simulink model "RBD_Adjoint"  (R2022a)
settings: Solver=ode4  StartTime=0.0  StopTime=10  FixedStep=0.001  MaxStep=0.01  RelTol=1e-3
model workspace (MAT data in the model file):
  D = 2
  K = 2
  X_d = [5; 5; 5]
values from neighbouring files (symbols this model uses):
  Ic = 2.0 0.0 0.0 0.0 5.0 0.0 0.0 0.0 8.0    [dictionary.sldd]
  m = 2.0    [dictionary.sldd]
  v_0 = 2.0 0.0 0.0    [dictionary.sldd]
  w_0 = 0.0 0.0 0.0    [dictionary.sldd]
settings Model: DataDictionary=dictionary.sldd  Creator=Tommaso  LastModifiedBy=Tommaso
settings OptimizationCC: DefaultParameterBehavior=Inlined  UseDivisionForNetSlopeComputation=on  GainParamInheritBuiltInType=on  UseFloatMulNetSlope=on  InlineInvariantSignals=on  PassReuseOutputArgsThreshold=0  ZeroExternalMemoryAtStartup=off  ZeroInternalMemoryAtStartup=off  EfficientFloat2IntCast=on  OptimizeBlockOrder=speed  DifferentSizesBufferReuse=on
settings DebuggingCC: ParameterTunabilityLossMsg=error  BusObjectLabelMismatch=error
settings SFSimCC: MATLABDynamicMemAlloc=off
settings RTWCC: Description=Generic Real-Time Target  GenerateReport=on  LaunchReport=on  TargetLang=C++
settings CodeAppCC: ForceParamTrailComments=on  OperatorAnnotations=on
settings GRTTargetCC: TargetLangStandard=C++11 (ISO)  CodeInterfacePackaging=C++ class  MultiInstanceErrorCode=Warning

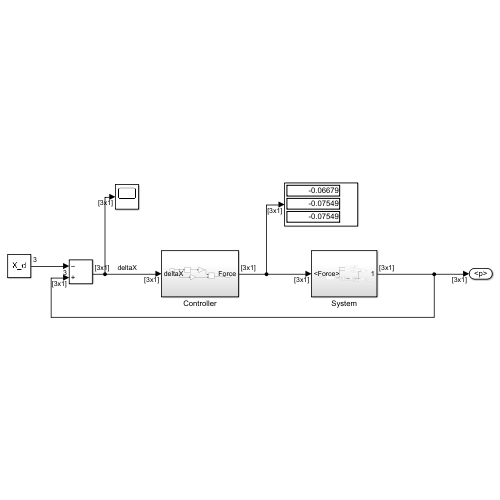
[thumbnail: Simulink's stored preview of the top-level diagram]
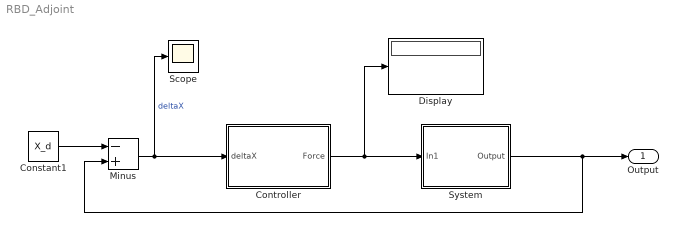
== system RBD_Adjoint ==
  Constant1 : Constant  Value=X_d
  Controller : Subsystem
  Display : Display
  Minus : Sum  Inputs=-+
  Scope : Scope
  System : Subsystem
  Output : Outport
  wires:
  System/1(Output) -> Output/1, Minus/2
  Constant1/1 -> Minus/1
  Minus/1 -> Controller/1(deltaX), Scope/1  "deltaX"
  Controller/1(Force) -> System/1(In1), Display/1

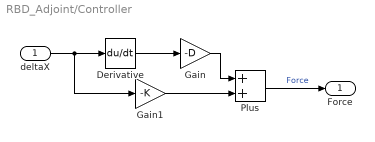
== system RBD_Adjoint/Controller ==
  deltaX : Inport
  Derivative : Derivative
  Gain : Gain  Gain=-D
  Gain1 : Gain  Gain=-K
  Plus : Sum
  Force : Outport
  wires:
  Derivative/1 -> Gain/1
  Gain1/1 -> Plus/2
  Gain/1 -> Plus/1
  Plus/1 -> Force/1  "Force"
  deltaX/1 -> Gain1/1, Derivative/1

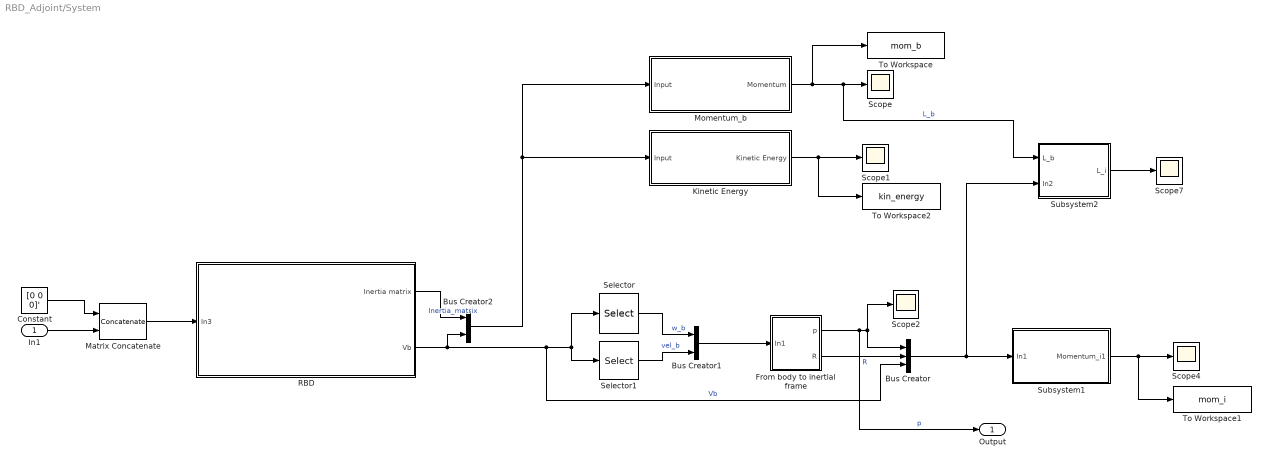
== system RBD_Adjoint/System ==
  In1 : Inport
  Bus Creator : BusCreator  Inputs=3  OutDataTypeStr=Bus: R_p_Vb
  Bus Creator1 : BusCreator  Inputs=2  OutDataTypeStr=Bus: Vb_bus  NonVirtualBus=on
  Bus Creator2 : BusCreator  Inputs=2  OutDataTypeStr=Bus: Inertia_Vb
  Constant : Constant  Value=[0 0 0]'
  From body to inertial frame : Subsystem  TreatAsAtomicUnit=on
  Kinetic Energy : Subsystem  TreatAsAtomicUnit=on
  Matrix Concatenate : Concatenate  Mode=Multidimensional array
  Momentum_b : Subsystem  TreatAsAtomicUnit=on
  RBD : Subsystem  TreatAsAtomicUnit=on
  Scope{,1..2,4,7} (5 alike) : Scope
  Selector : Selector  InputPortWidth=6  IndexOptions=Index vector (dialog)  Indices=[1,2,3]  OutputSizes=1
  Selector1 : Selector  InputPortWidth=6  IndexOptions=Index vector (dialog)  Indices=[4:6]  OutputSizes=1
  Subsystem1 : Subsystem  TreatAsAtomicUnit=on
  Subsystem2 : Subsystem  TreatAsAtomicUnit=on
  To Workspace : ToWorkspace  VariableName=mom_b  SampleTime=-1
  To Workspace1 : ToWorkspace  VariableName=mom_i  SampleTime=-1
  To Workspace2 : ToWorkspace  VariableName=kin_energy  SampleTime=-1
  Output : Outport
  wires:
  Subsystem1/1(Momentum_i1) -> To Workspace1/1, Scope4/1
  Bus Creator/1 -> Subsystem1/1(In1), Subsystem2/2(In2)
  Momentum_b/1(Momentum) -> To Workspace/1, Subsystem2/1(L_b), Scope/1  "L_b"
  Selector/1 -> Bus Creator1/1  "w_b"
  Kinetic Energy/1(Kinetic Energy) -> To Workspace2/1, Scope1/1
  RBD/1(Inertia matrix) -> Bus Creator2/1  "Inertia_matrix"
  Bus Creator2/1 -> Momentum_b/1(Input), Kinetic Energy/1(Input)
  Selector1/1 -> Bus Creator1/2  "vel_b"
  RBD/2(Vb) -> Bus Creator2/2, Bus Creator/3, Selector/1, Selector1/1  "Vb"
  Bus Creator1/1 -> From body to inertial frame/1(In1)
  From body to inertial frame/1(p) -> Output/1, Bus Creator/1, Scope2/1  "p"
  From body to inertial frame/2(R) -> Bus Creator/2  "R"
  Subsystem2/1(L_i) -> Scope7/1
  In1/1 -> Matrix Concatenate/2
  Matrix Concatenate/1 -> RBD/1(In3)
  Constant/1 -> Matrix Concatenate/1

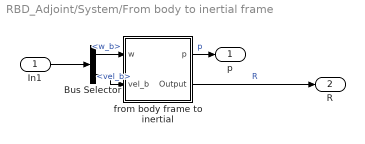
== system RBD_Adjoint/System/From body to inertial frame ==
  In1 : Inport
  Bus Selector : BusSelector  OutputSignals=w_b,vel_b
  from body frame to inertial : Subsystem
  p : Outport
  R : Outport  Port=2
  wires:
  Bus Selector/1 -> from body frame to inertial/1(w)  "<w_b>"
  from body frame to inertial/2(Output) -> R/1  "R"
  Bus Selector/2 -> from body frame to inertial/2(vel_b)  "<vel_b>"
  from body frame to inertial/1(p) -> p/1  "p"
  In1/1 -> Bus Selector/1

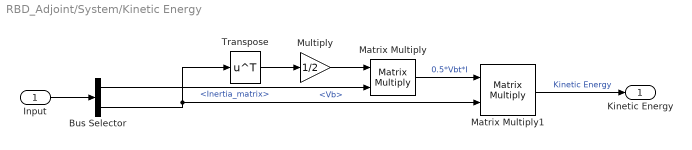
== system RBD_Adjoint/System/Kinetic Energy ==
  Input : Inport
  Bus Selector : BusSelector  OutputSignals=Inertia_matrix,Vb
  Matrix Multiply : Product  Multiplication=Matrix(*)
  Matrix Multiply1 : Product  Multiplication=Matrix(*)
  Multiply : Gain  Gain=1/2
  Transpose : Math  Operator=transpose
  Kinetic Energy : Outport
  wires:
  Bus Selector/2 -> Matrix Multiply1/2, Transpose/1  "<Vb>"
  Multiply/1 -> Matrix Multiply/1
  Transpose/1 -> Multiply/1
  Matrix Multiply/1 -> Matrix Multiply1/1  "0.5*Vbt*I"
  Matrix Multiply1/1 -> Kinetic Energy/1  "Kinetic Energy"
  Input/1 -> Bus Selector/1
  Bus Selector/1 -> Matrix Multiply/2  "<Inertia_matrix>"

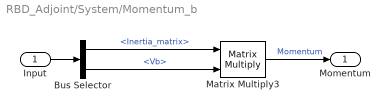
== system RBD_Adjoint/System/Momentum_b ==
  Input : Inport
  Bus Selector : BusSelector  OutputSignals=Inertia_matrix,Vb
  Matrix Multiply3 : Product  Multiplication=Matrix(*)
  Momentum : Outport
  wires:
  Matrix Multiply3/1 -> Momentum/1  "Momentum"
  Bus Selector/1 -> Matrix Multiply3/1  "<Inertia_matrix>"
  Input/1 -> Bus Selector/1
  Bus Selector/2 -> Matrix Multiply3/2  "<Vb>"

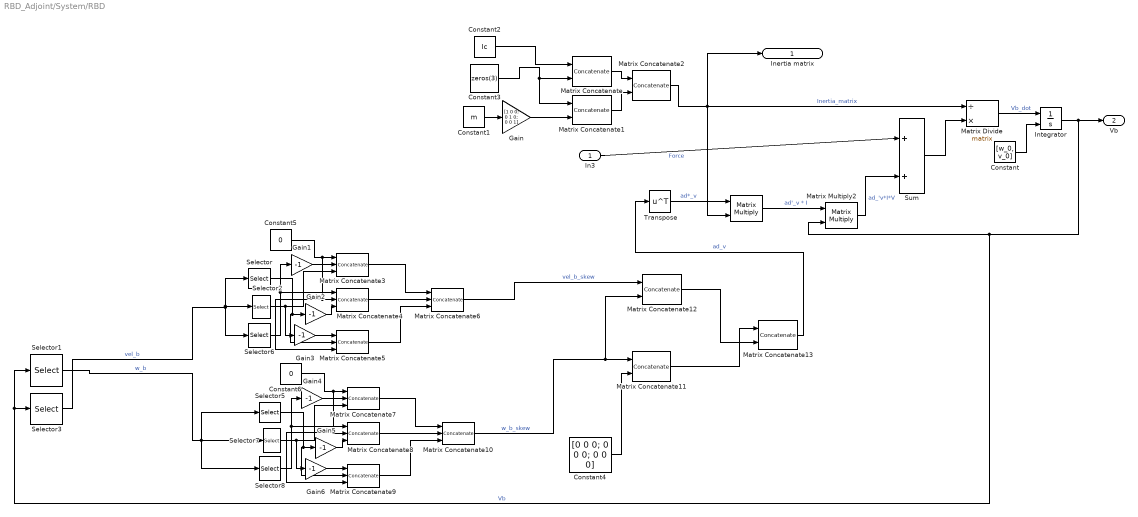
== system RBD_Adjoint/System/RBD ==
  In3 : Inport
  " " : Product  Multiplication=Matrix(*)
  Constant : Constant  Value=[w_0, v_0]
  Constant1 : Constant  Value=m
  Constant2 : Constant  Value=Ic
  Constant3 : Constant  Value=zeros(3)
  Constant4 : Constant  Value=[0 0 0; 0 0 0; 0 0 0]
  Constant5 : Constant  Value=0
  Constant6 : Constant  Value=0
  Gain : Gain  Gain=[1 0 0; 0 1 0; 0 0 1]
  Gain{1..6} (6 alike) : Gain  Gain=-1
  Integrator : Integrator  InitialConditionSource=external
  Matrix Concatenate{,1,11..12} (4 alike) : Concatenate  Mode=Multidimensional array  ConcatenateDimension=2
  Matrix Concatenate10 : Concatenate  NumInputs=3  Mode=Multidimensional array
  Matrix Concatenate13 : Concatenate  Mode=Multidimensional array
  Matrix Concatenate2 : Concatenate  Mode=Multidimensional array
  Matrix Concatenate{3..5,7..9} (6 alike) : Concatenate  NumInputs=3  Mode=Multidimensional array  ConcatenateDimension=2
  Matrix Concatenate6 : Concatenate  NumInputs=3  Mode=Multidimensional array
  Matrix Divide : Product  Inputs=/*  Multiplication=Matrix(*)
  Matrix Multiply2 : Product  Multiplication=Matrix(*)
  Selector : Selector  InputPortWidth=3  IndexOptions=Index vector (dialog)  Indices=1  OutputSizes=1
  Selector1 : Selector  InputPortWidth=6  IndexOptions=Index vector (dialog)  Indices=[1,2,3]  OutputSizes=1
  Selector2 : Selector  InputPortWidth=3  IndexOptions=Index vector (dialog)  Indices=2  OutputSizes=1
  Selector3 : Selector  InputPortWidth=6  IndexOptions=Index vector (dialog)  Indices=[4:6]  OutputSizes=1
  Selector5 : Selector  InputPortWidth=3  IndexOptions=Index vector (dialog)  Indices=1  OutputSizes=1
  Selector6 : Selector  InputPortWidth=3  IndexOptions=Index vector (dialog)  Indices=3  OutputSizes=1
  Selector7 : Selector  InputPortWidth=3  IndexOptions=Index vector (dialog)  Indices=2  OutputSizes=1
  Selector8 : Selector  InputPortWidth=3  IndexOptions=Index vector (dialog)  Indices=3  OutputSizes=1
  Sum : Sum  Inputs=|++
  Transpose : Math  Operator=transpose
  Inertia matrix : Outport
  Vb : Outport  Port=2
  wires:
  Integrator/1 -> Selector1/1, Selector3/1, Matrix Multiply2/2, Vb/1  "Vb"
  Matrix Multiply2/1 -> Sum/2  "ad_'v*I*V"
  " "/1 -> Matrix Multiply2/1  "ad'_v * I"
  Matrix Divide/1 -> Integrator/1  "Vb_dot"
  Matrix Concatenate2/1 -> " "/2, Inertia matrix/1, Matrix Divide/1  "Inertia_matrix"
  Transpose/1 -> " "/1  "ad*_v"
  Sum/1 -> Matrix Divide/2
  Constant1/1 -> Gain/1
  Constant2/1 -> Matrix Concatenate/1
  In3/1 -> Sum/1  "Force"
  Constant/1 -> Integrator/2
  Constant3/1 -> Matrix Concatenate1/1, Matrix Concatenate/2
  Gain/1 -> Matrix Concatenate1/2
  Matrix Concatenate/1 -> Matrix Concatenate2/1
  Matrix Concatenate1/1 -> Matrix Concatenate2/2
  Constant5/1 -> Matrix Concatenate5/3, Matrix Concatenate4/2, Matrix Concatenate3/1
  Selector2/1 -> Gain3/1, Matrix Concatenate3/3
  Selector6/1 -> Matrix Concatenate4/1, Gain1/1
  Gain1/1 -> Matrix Concatenate3/2
  Matrix Concatenate3/1 -> Matrix Concatenate6/1
  Selector/1 -> Gain2/1, Matrix Concatenate5/2
  Gain2/1 -> Matrix Concatenate4/3
  Matrix Concatenate4/1 -> Matrix Concatenate6/2
  Gain3/1 -> Matrix Concatenate5/1
  Matrix Concatenate5/1 -> Matrix Concatenate6/3
  Matrix Concatenate6/1 -> Matrix Concatenate12/1  "vel_b_skew"
  Selector5/1 -> Gain5/1, Matrix Concatenate9/2
  Gain5/1 -> Matrix Concatenate8/3
  Selector7/1 -> Gain6/1, Matrix Concatenate7/3
  Matrix Concatenate7/1 -> Matrix Concatenate10/1
  Matrix Concatenate9/1 -> Matrix Concatenate10/3
  Gain4/1 -> Matrix Concatenate7/2
  Selector8/1 -> Matrix Concatenate8/1, Gain4/1
  Matrix Concatenate8/1 -> Matrix Concatenate10/2
  Gain6/1 -> Matrix Concatenate9/1
  Constant6/1 -> Matrix Concatenate9/3, Matrix Concatenate8/2, Matrix Concatenate7/1
  Matrix Concatenate10/1 -> Matrix Concatenate12/2, Matrix Concatenate11/1  "w_b_skew"
  Constant4/1 -> Matrix Concatenate11/2
  Matrix Concatenate12/1 -> Matrix Concatenate13/2
  Matrix Concatenate11/1 -> Matrix Concatenate13/1
  Matrix Concatenate13/1 -> Transpose/1  "ad_v"
  Selector1/1 -> Selector5/1, Selector8/1, Selector7/1  "w_b"
  Selector3/1 -> Selector6/1, Selector/1, Selector2/1  "vel_b"

== system RBD_Adjoint/System/Subsystem1 ==
  In1 : Inport
  Bus Selector : BusSelector  OutputSignals=p,R,Vb
  Momentum_i : Subsystem
  Momentum_i1 : Outport
  wires:
  Bus Selector/1 -> Momentum_i/1(p)  "<p>"
  In1/1 -> Bus Selector/1
  Bus Selector/3 -> Momentum_i/3(Vb)  "<Vb>"
  Bus Selector/2 -> Momentum_i/2(R)  "<R>"
  Momentum_i/1(Momentum_i) -> Momentum_i1/1

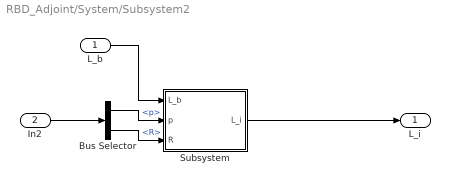
== system RBD_Adjoint/System/Subsystem2 ==
  L_b : Inport
  In2 : Inport  Port=2
  Bus Selector : BusSelector  OutputSignals=p,R
  Subsystem : Subsystem
  L_i : Outport
  wires:
  L_b/1 -> Subsystem/1(L_b)
  Bus Selector/2 -> Subsystem/3(R)  "<R>"
  Bus Selector/1 -> Subsystem/2(p)  "<p>"
  In2/1 -> Bus Selector/1
  Subsystem/1(L_i) -> L_i/1

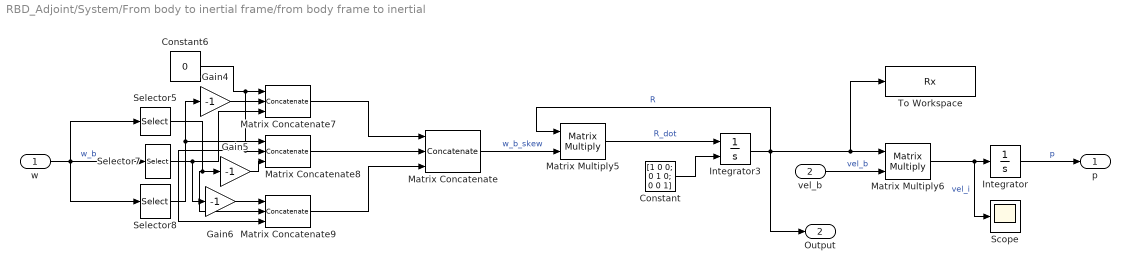
== system RBD_Adjoint/System/From body to inertial frame/from body frame to inertial ==
  w : Inport
  vel_b : Inport  Port=2
  Constant : Constant  Value=[1 0 0; 0 1 0; 0 0 1]
  Constant6 : Constant  Value=0
  Gain4 : Gain  Gain=-1
  Gain5 : Gain  Gain=-1
  Gain6 : Gain  Gain=-1
  Integrator : Integrator
  Integrator3 : Integrator  InitialConditionSource=external
  Matrix Concatenate : Concatenate  NumInputs=3  Mode=Multidimensional array
  Matrix Concatenate7 : Concatenate  NumInputs=3  Mode=Multidimensional array  ConcatenateDimension=2
  Matrix Concatenate8 : Concatenate  NumInputs=3  Mode=Multidimensional array  ConcatenateDimension=2
  Matrix Concatenate9 : Concatenate  NumInputs=3  Mode=Multidimensional array  ConcatenateDimension=2
  Matrix Multiply5 : Product  Multiplication=Matrix(*)
  Matrix Multiply6 : Product  Multiplication=Matrix(*)
  Scope : Scope
  Selector5 : Selector  InputPortWidth=3  IndexOptions=Index vector (dialog)  Indices=1  OutputSizes=1
  Selector7 : Selector  InputPortWidth=3  IndexOptions=Index vector (dialog)  Indices=2  OutputSizes=1
  Selector8 : Selector  InputPortWidth=3  IndexOptions=Index vector (dialog)  Indices=3  OutputSizes=1
  To Workspace : ToWorkspace  VariableName=Rx  SaveFormat=Structure With Time  SampleTime=-1
  p : Outport
  Output : Outport  Port=2
  wires:
  Integrator3/1 -> Output/1, To Workspace/1, Matrix Multiply6/1, Matrix Multiply5/1  "R"
  Matrix Multiply5/1 -> Integrator3/1  "R_dot"
  Matrix Concatenate/1 -> Matrix Multiply5/2  "w_b_skew"
  vel_b/1 -> Matrix Multiply6/2  "vel_b"
  Matrix Multiply6/1 -> Scope/1, Integrator/1  "vel_i"
  Integrator/1 -> p/1  "p"
  Constant/1 -> Integrator3/2
  Selector5/1 -> Gain5/1, Matrix Concatenate9/2
  Selector7/1 -> Gain6/1, Matrix Concatenate7/3
  Gain6/1 -> Matrix Concatenate9/1
  Matrix Concatenate8/1 -> Matrix Concatenate/2
  Gain4/1 -> Matrix Concatenate7/2
  Gain5/1 -> Matrix Concatenate8/3
  Matrix Concatenate7/1 -> Matrix Concatenate/1
  Selector8/1 -> Matrix Concatenate8/1, Gain4/1
  Matrix Concatenate9/1 -> Matrix Concatenate/3
  w/1 -> Selector8/1, Selector5/1, Selector7/1  "w_b"
  Constant6/1 -> Matrix Concatenate9/3, Matrix Concatenate8/2, Matrix Concatenate7/1

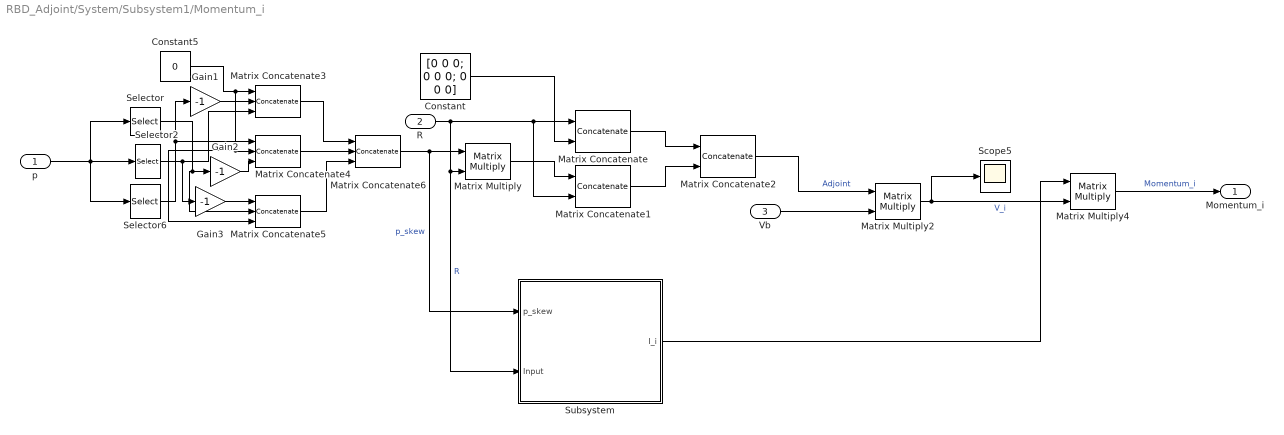
== system RBD_Adjoint/System/Subsystem1/Momentum_i ==
  p : Inport
  R : Inport  Port=2
  Vb : Inport  Port=3
  Constant : Constant  Value=[0 0 0; 0 0 0; 0 0 0]
  Constant5 : Constant  Value=0
  Gain1 : Gain  Gain=-1
  Gain2 : Gain  Gain=-1
  Gain3 : Gain  Gain=-1
  Matrix Concatenate : Concatenate  Mode=Multidimensional array  ConcatenateDimension=2
  Matrix Concatenate1 : Concatenate  Mode=Multidimensional array  ConcatenateDimension=2
  Matrix Concatenate2 : Concatenate  Mode=Multidimensional array
  Matrix Concatenate3 : Concatenate  NumInputs=3  Mode=Multidimensional array  ConcatenateDimension=2
  Matrix Concatenate4 : Concatenate  NumInputs=3  Mode=Multidimensional array  ConcatenateDimension=2
  Matrix Concatenate5 : Concatenate  NumInputs=3  Mode=Multidimensional array  ConcatenateDimension=2
  Matrix Concatenate6 : Concatenate  NumInputs=3  Mode=Multidimensional array
  Matrix Multiply : Product  Multiplication=Matrix(*)
  Matrix Multiply2 : Product  Multiplication=Matrix(*)
  Matrix Multiply4 : Product  Multiplication=Matrix(*)
  Scope5 : Scope
  Selector : Selector  InputPortWidth=3  IndexOptions=Index vector (dialog)  Indices=1  OutputSizes=1
  Selector2 : Selector  InputPortWidth=3  IndexOptions=Index vector (dialog)  Indices=2  OutputSizes=1
  Selector6 : Selector  InputPortWidth=3  IndexOptions=Index vector (dialog)  Indices=3  OutputSizes=1
  Subsystem : Subsystem
  Momentum_i : Outport
  wires:
  Matrix Multiply2/1 -> Matrix Multiply4/2, Scope5/1  "V_i"
  R/1 -> Matrix Concatenate1/2, Matrix Concatenate/1, Subsystem/2(Input), Matrix Multiply/2  "R"
  Vb/1 -> Matrix Multiply2/2
  Matrix Multiply4/1 -> Momentum_i/1  "Momentum_i"
  Matrix Concatenate2/1 -> Matrix Multiply2/1  "Adjoint"
  Selector/1 -> Gain2/1, Matrix Concatenate5/2
  Gain2/1 -> Matrix Concatenate4/3
  Selector2/1 -> Gain3/1, Matrix Concatenate3/3
  Matrix Concatenate3/1 -> Matrix Concatenate6/1
  Matrix Concatenate5/1 -> Matrix Concatenate6/3
  p/1 -> Selector2/1, Selector6/1, Selector/1
  Gain1/1 -> Matrix Concatenate3/2
  Selector6/1 -> Matrix Concatenate4/1, Gain1/1
  Matrix Concatenate4/1 -> Matrix Concatenate6/2
  Gain3/1 -> Matrix Concatenate5/1
  Constant5/1 -> Matrix Concatenate5/3, Matrix Concatenate4/2, Matrix Concatenate3/1
  Matrix Concatenate6/1 -> Subsystem/1(p_skew), Matrix Multiply/1  "p_skew"
  Constant/1 -> Matrix Concatenate/2
  Matrix Multiply/1 -> Matrix Concatenate1/1
  Matrix Concatenate/1 -> Matrix Concatenate2/1
  Matrix Concatenate1/1 -> Matrix Concatenate2/2
  Subsystem/1(I_i) -> Matrix Multiply4/1

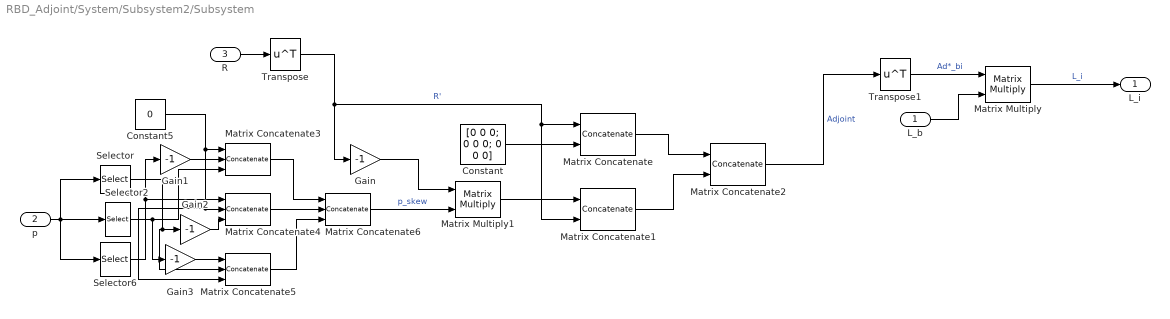
== system RBD_Adjoint/System/Subsystem2/Subsystem ==
  L_b : Inport
  p : Inport  Port=2
  R : Inport  Port=3
  Constant : Constant  Value=[0 0 0; 0 0 0; 0 0 0]
  Constant5 : Constant  Value=0
  Gain{,1..3} (4 alike) : Gain  Gain=-1
  Matrix Concatenate : Concatenate  Mode=Multidimensional array  ConcatenateDimension=2
  Matrix Concatenate1 : Concatenate  Mode=Multidimensional array  ConcatenateDimension=2
  Matrix Concatenate2 : Concatenate  Mode=Multidimensional array
  Matrix Concatenate3 : Concatenate  NumInputs=3  Mode=Multidimensional array  ConcatenateDimension=2
  Matrix Concatenate4 : Concatenate  NumInputs=3  Mode=Multidimensional array  ConcatenateDimension=2
  Matrix Concatenate5 : Concatenate  NumInputs=3  Mode=Multidimensional array  ConcatenateDimension=2
  Matrix Concatenate6 : Concatenate  NumInputs=3  Mode=Multidimensional array
  Matrix Multiply : Product  Multiplication=Matrix(*)
  Matrix Multiply1 : Product  Multiplication=Matrix(*)
  Selector : Selector  InputPortWidth=3  IndexOptions=Index vector (dialog)  Indices=1  OutputSizes=1
  Selector2 : Selector  InputPortWidth=3  IndexOptions=Index vector (dialog)  Indices=2  OutputSizes=1
  Selector6 : Selector  InputPortWidth=3  IndexOptions=Index vector (dialog)  Indices=3  OutputSizes=1
  Transpose : Math  Operator=transpose
  Transpose1 : Math  Operator=transpose
  L_i : Outport
  wires:
  Transpose1/1 -> Matrix Multiply/1  "Ad*_bi"
  L_b/1 -> Matrix Multiply/2
  Matrix Multiply/1 -> L_i/1  "L_i"
  Gain1/1 -> Matrix Concatenate3/2
  Matrix Concatenate4/1 -> Matrix Concatenate6/2
  Selector6/1 -> Matrix Concatenate4/1, Gain1/1
  Matrix Concatenate5/1 -> Matrix Concatenate6/3
  Gain2/1 -> Matrix Concatenate4/3
  Matrix Concatenate3/1 -> Matrix Concatenate6/1
  Gain3/1 -> Matrix Concatenate5/1
  Constant5/1 -> Matrix Concatenate5/3, Matrix Concatenate4/2, Matrix Concatenate3/1
  Selector/1 -> Gain2/1, Matrix Concatenate5/2
  Selector2/1 -> Gain3/1, Matrix Concatenate3/3
  p/1 -> Selector2/1, Selector6/1, Selector/1
  Matrix Concatenate6/1 -> Matrix Multiply1/2  "p_skew"
  R/1 -> Transpose/1
  Transpose/1 -> Gain/1, Matrix Concatenate1/2, Matrix Concatenate/1  "R'"
  Constant/1 -> Matrix Concatenate/2
  Gain/1 -> Matrix Multiply1/1
  Matrix Multiply1/1 -> Matrix Concatenate1/1
  Matrix Concatenate/1 -> Matrix Concatenate2/1
  Matrix Concatenate1/1 -> Matrix Concatenate2/2
  Matrix Concatenate2/1 -> Transpose1/1  "Adjoint"

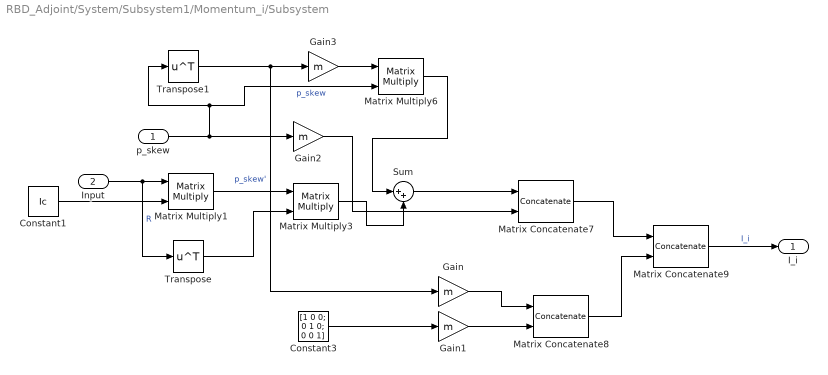
== system RBD_Adjoint/System/Subsystem1/Momentum_i/Subsystem ==
  p_skew : Inport
  Input : Inport  Port=2
  Constant1 : Constant  Value=Ic
  Constant3 : Constant  Value=[1 0 0; 0 1 0; 0 0 1]
  Gain{,1..3} (4 alike) : Gain  Gain=m
  Matrix Concatenate7 : Concatenate  Mode=Multidimensional array  ConcatenateDimension=2
  Matrix Concatenate8 : Concatenate  Mode=Multidimensional array  ConcatenateDimension=2
  Matrix Concatenate9 : Concatenate  Mode=Multidimensional array
  Matrix Multiply1 : Product  Multiplication=Matrix(*)
  Matrix Multiply3 : Product  Multiplication=Matrix(*)
  Matrix Multiply6 : Product  Multiplication=Matrix(*)
  Sum : Sum  Inputs=|++
  Transpose : Math  Operator=transpose
  Transpose1 : Math  Operator=transpose
  I_i : Outport
  wires:
  p_skew/1 -> Gain2/1, Matrix Multiply6/2, Transpose1/1  "p_skew"
  Transpose/1 -> Matrix Multiply3/2
  Matrix Concatenate7/1 -> Matrix Concatenate9/1
  Input/1 -> Transpose/1, Matrix Multiply1/1  "R"
  Transpose1/1 -> Gain3/1, Gain/1  "p_skew'"
  Matrix Multiply3/1 -> Sum/2
  Gain3/1 -> Matrix Multiply6/1
  Sum/1 -> Matrix Concatenate7/1
  Matrix Multiply6/1 -> Sum/1
  Gain2/1 -> Matrix Concatenate7/2
  Constant1/1 -> Matrix Multiply1/2
  Gain/1 -> Matrix Concatenate8/1
  Matrix Multiply1/1 -> Matrix Multiply3/1
  Matrix Concatenate8/1 -> Matrix Concatenate9/2
  Matrix Concatenate9/1 -> I_i/1  "I_i"
  Constant3/1 -> Gain1/1
  Gain1/1 -> Matrix Concatenate8/2
